simulink model "obsver_k"  (R2013a)
settings: Solver=ode45  StartTime=0.0  StopTime=20  RelTol=1e-3
values from neighbouring files (symbols this model uses):
  A = [S3 S6 S7;S6 S8 S9; S7 S9 S10]    [LSQ_regression.m]
  G = acker(A',C',P1)'    [adapt_compute.m]
undefined symbols (not defined in the file or in its folder): C
settings Model: Creator=Aleksandr  LastModifiedBy=Aleksandr

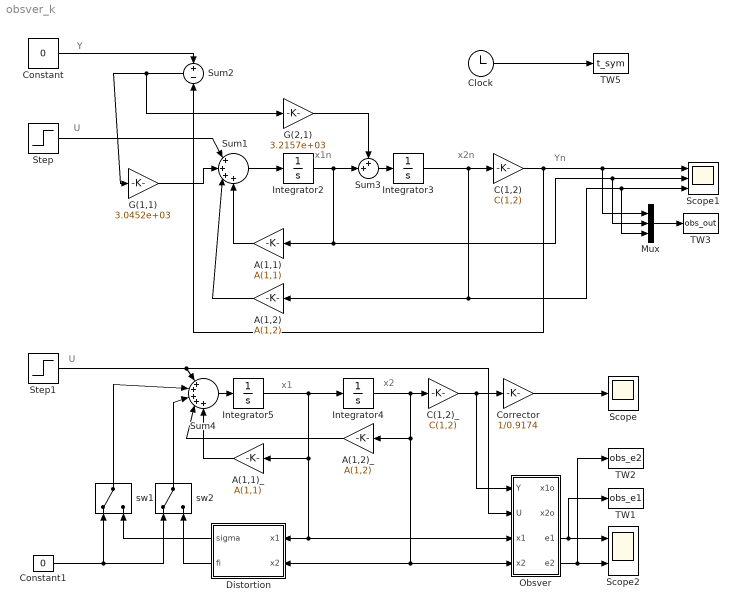
== system obsver_k ==
  note: U
  note: Yn
  note: U
  note: Y
  note: x1n
  note: x2n
  note: x2
  note: x1
  A(1,1) : Gain  Gain=A(1,1)
  A(1,1)_ : Gain  Gain=A(1,1)
  A(1,2) : Gain  Gain=A(1,2)
  A(1,2)_ : Gain  Gain=A(1,2)
  C(1,2) : Gain  Gain=C(1,2)
  C(1,2)_ : Gain  Gain=C(1,2)
  Clock : Clock
      settings: Decimation=2000
  Constant : Constant  Value=0
  Constant1 : Constant  Value=0
  Corrector : Gain  Gain=1/0.9174
  Distortion : Subsystem
  G(1,1) : Gain  Gain=3.0452e+03
  G(2,1) : Gain  Gain=3.2157e+03
  Integrator{2..5} (4 alike) : Integrator
  Mux : Mux  Inputs=3
  Obsver : Subsystem
  Scope : Scope
  Scope1 : Scope  NumInputPorts=3
      settings: TimeRange=2000  YMin=-0.01~-5~-5  YMax=0~5~5
  Scope2 : Scope  NumInputPorts=2
      settings: YMin=-5~-5  YMax=5~5  SaveName=ScopeData2
  Step : Step  Time=0  SampleTime=0
  Step1 : Step  Time=0  SampleTime=0
  Sum1 : Sum  Inputs=|++++
  Sum2 : Sum  Inputs=+-
  Sum3 : Sum  Inputs=++|
  Sum4 : Sum  Inputs=|+++++
  TW1 : ToWorkspace  VariableName=obs_e1  SampleTime=-1
  TW2 : ToWorkspace  VariableName=obs_e2  SampleTime=-1
  TW3 : ToWorkspace  VariableName=obs_out  SampleTime=-1
  TW5 : ToWorkspace  VariableName=t_sym  SampleTime=-1
  sw1 : ManualSwitch
  sw2 : ManualSwitch
  wires:
  Integrator3/1 -> C(1,2)/1, A(1,2)/1, Mux/3, Scope1/3
  Integrator2/1 -> A(1,1)/1, Mux/2, Scope1/2, Sum3/2
  Sum1/1 -> Integrator2/1
  Step/1 -> Sum1/1
  A(1,1)/1 -> Sum1/4
  Constant/1 -> Sum2/1
  Sum3/1 -> Integrator3/1
  Sum2/1 -> G(1,1)/1, G(2,1)/1
  G(2,1)/1 -> Sum3/1
  G(1,1)/1 -> Sum1/2
  A(1,2)/1 -> Sum1/3
  C(1,2)/1 -> Mux/1, Scope1/1, Sum2/2
  C(1,2)_/1 -> Obsver/1(Y), Corrector/1
  Sum4/1 -> Integrator5/1
  Integrator4/1 -> Distortion/2(x2), Obsver/4(x2), A(1,2)_/1, C(1,2)_/1
  Integrator5/1 -> Obsver/3(x1), Distortion/1(x1), A(1,1)_/1, Integrator4/1
  A(1,1)_/1 -> Sum4/5
  A(1,2)_/1 -> Sum4/4
  Distortion/1(sigma) -> sw1/2
  Distortion/2(fi) -> sw2/2
  Constant1/1 -> sw1/1, sw2/1
  sw2/1 -> Sum4/3
  sw1/1 -> Sum4/2
  Corrector/1 -> Scope/1
  Obsver/3(e1) -> TW1/1, Scope2/1
  Obsver/4(e2) -> TW2/1, Scope2/2
  Clock/1 -> TW5/1
  Mux/1 -> TW3/1
  Step1/1 -> Sum4/1, Obsver/2(U)

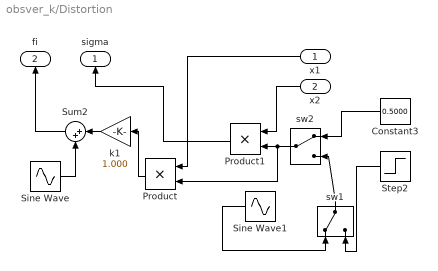
== system obsver_k/Distortion ==
  x1 : Inport
  x2 : Inport  Port=2
  Constant3 : Constant  Value=0.5000
  Product : Product
  Product1 : Product
  Sine Wave : Sin  Frequency=pi/2  SampleTime=0
  Sine Wave1 : Sin  SampleTime=0
  Step2 : Step  Time=0  After=0.5  SampleTime=0
  Sum2 : Sum  Inputs=|++
  k1 : Gain  Gain=1.000
  sw1 : ManualSwitch
  sw2 : ManualSwitch
  sigma : Outport
  fi : Outport  Port=2
  wires:
  x1/1 -> Product/1
  Product1/1 -> sigma/1
  Sum2/1 -> fi/1
  x2/1 -> Product1/1
  sw2/1 -> Product/2, Product1/2
  Step2/1 -> sw1/2
  Product/1 -> k1/1
  k1/1 -> Sum2/1
  Sine Wave/1 -> Sum2/2
  Constant3/1 -> sw2/1
  sw1/1 -> sw2/2
  Sine Wave1/1 -> sw1/1

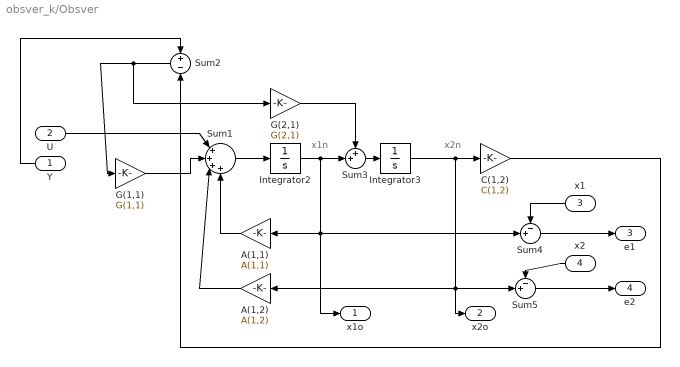
== system obsver_k/Obsver ==
  note: x1n
  note: x2n
  Y : Inport
  U : Inport  Port=2
  x1 : Inport  Port=3
  x2 : Inport  Port=4
  A(1,1) : Gain  Gain=A(1,1)
  A(1,2) : Gain  Gain=A(1,2)
  C(1,2) : Gain  Gain=C(1,2)
  G(1,1) : Gain  Gain=G(1,1)
  G(2,1) : Gain  Gain=G(2,1)
  Integrator2 : Integrator
  Integrator3 : Integrator
  Sum1 : Sum  Inputs=|++++
  Sum2 : Sum  Inputs=+-
  Sum3 : Sum  Inputs=++|
  Sum4 : Sum  Inputs=-+|
  Sum5 : Sum  Inputs=-+|
  x1o : Outport
  x2o : Outport  Port=2
  e1 : Outport  Port=3
  e2 : Outport  Port=4
  wires:
  C(1,2)/1 -> Sum2/2
  x2/1 -> Sum5/1
  Integrator2/1 -> A(1,1)/1, Sum4/2, x1o/1, Sum3/2
  Sum1/1 -> Integrator2/1
  U/1 -> Sum1/1
  A(1,1)/1 -> Sum1/4
  Y/1 -> Sum2/1
  x1/1 -> Sum4/1
  Sum5/1 -> e2/1
  Sum3/1 -> Integrator3/1
  Sum4/1 -> e1/1
  Sum2/1 -> G(1,1)/1, G(2,1)/1
  G(2,1)/1 -> Sum3/1
  G(1,1)/1 -> Sum1/2
  A(1,2)/1 -> Sum1/3
  Integrator3/1 -> C(1,2)/1, Sum5/2, A(1,2)/1, x2o/1
